simulink library "formationFlyingBlockset"  (R2016b)
settings: Solver=ode45  StartTime=0.0  StopTime=10.0  RelTol=1e-3  EnableMultiTasking=on
undefined symbols (not defined in the file or in its folder): adaptive, aircraftmask_ID, aircraftmask_navigationLaw, aircraftmask_originNED_ECEF_rrm, aircraftmask_p0_NED_m, aircraftmask_phithetapsi_trim, aircraftmask_wakevortexenabled, airkraftmask_displayLeader, DiscIntNeverNeededParam, Earth, fflib_degdegm2rrm, fflib_Hz2radps, fflib_rrm2degdegm, flat2lla, hinf, Klqr, lquadr, mask_ac, mask_ID, mpc, poleplacement, uavsim, washout, WGS84
undefined symbols (not defined in the file): aircraftmask_phithetapsi0, aircraftmask_pqr0, aircraftmask_uvw0, innerloop, outerloop, tatestos
libraries: formationFlyingBlockset x59, aerolibtransform2 x42, simulink_extras x27, dspsrcs4 x11, aerolibutil x5, uavsimBlockset_UAV3DInterface x4, uavsimBlockset_ServoHS55 x4, uavsimBlockset_VectorNorm x3, uavsimBlockset_UAV3DVisualization x3, uavsimBlockset_AugmentWind x3, stringquartett x2, Parrot_DCAS_lib x2
(part 2 of 5)

== system formationFlyingBlockset/Parrot drone ==
  Environment : Inport  OutDataTypeStr=Bus: Environment
  Bus Creator : BusCreator  Inputs=2  OutDataTypeStr=Bus: iUAScom
  Bus Creator1 : BusCreator  Inputs=1  OutDataTypeStr=Bus: FlightGearData  NonVirtualBus=on
  Bus Selector1 : BusSelector  OutputSignals=Kinematics.Position.P_NED_m,Kinematics.Velocity.Vground_NED_mps
  Constant : Constant  Value=zeros(6,1)
  Gain : Gain
  Gain1 : Gain
  ID : Constant  Value=aircraftmask_ID
  MATLAB Function : MATLAB Function  TreatAsAtomicUnit=on
  No Elevation model : Constant  Value=0
  Parrot drone open loop dynamics : formationFlyingBlockset/Parrot drone open loop dynamics  mask_phithetapsi0=aircraftmask_phithetapsi0  mask_p0_ECEF_lla=fflib_degdegm2rrm(flat2lla(aircraftmask_p0_NED_m, rad2deg(aircraftmask_originNED_ECEF_rrm(1:2)), 0, aircraftmask_originNED_ECEF_rrm(3)))  mask_originNED_ECEF_rrm=aircraftmask_originNED_ECEF_rrm  mask_pqr0=aircraftmask_pqr0  mask_uvw0=aircraftmask_uvw0  uavsim=uavsim
  Simulation Time : formationFlyingBlockset/Signal to workspace  mask_id=['log_machinetime_UAS' num2str(aircraftmask_ID) ]  mask_dt=1  mask_debug=log_machinetime_UAS1
  Terminator5 : Terminator
  UAV3D Visualization : uavsimBlockset_UAV3DVisualization/UAV3D Visualization  mask_visual=3
  control surface deflections : formationFlyingBlockset/Signal to workspace  mask_id=['log_csdeflct_UAS' num2str(aircraftmask_ID) ]  mask_dt=-1  mask_debug=log_csdeflct_UAS1
  AirframeBus : Outport
  Grounddata : Outport  Port=2  OutDataTypeStr=Bus: FlightGearData
  iUASCom out : Outport  Port=3
  wires:
  MATLAB Function/1(t) -> Simulation Time/1
  Bus Creator/1 -> iUASCom out/1
  Bus Selector1/2 -> Gain/1  "<Vground_NED_mps>"
  Bus Selector1/1 -> Gain1/1  "<P_NED_m>"
  Gain1/1 -> Bus Creator/1  "P_NED_m"
  Gain/1 -> Bus Creator/2  "Vground_NED_mps"
  Constant/1 -> Parrot drone open loop dynamics/3
  Parrot drone open loop dynamics/3 -> control surface deflections/1, UAV3D Visualization/3
  Parrot drone open loop dynamics/1 -> Bus Selector1/1, AirframeBus/1, UAV3D Visualization/1
  Environment/1 -> Parrot drone open loop dynamics/2
  ID/1 -> UAV3D Visualization/2
  Bus Creator1/1 -> Grounddata/1
  No Elevation model/1 -> Bus Creator1/1  "groundlevel_NED_m"
  UAV3D Visualization/1 -> Terminator5/1

== system formationFlyingBlockset/Parrot drone open loop dynamics ==
  u - system inputs : Inport  OutDataTypeStr=Bus: CMD_quadrotor
  Environment : Inport  Port=2  OutDataTypeStr=Bus: Environment
  External forces and moments : Inport  Port=3
  Vehicle model : Subsystem
  Airframe : Outport  OutDataTypeStr=Bus: Airframe
  C_aero_w : Outport  Port=2
  effective commands : Outport  Port=3  OutDataTypeStr=Bus: CMD_quadrotor
  FMprop : Outport  Port=4
  wires:
  Environment/1 -> Vehicle model/2(EnvData)
  Vehicle model/2(Cwind) -> C_aero_w/1
  External forces and moments/1 -> Vehicle model/3(FM_external)
  u - system inputs/1 -> Vehicle model/1(CMD), effective commands/1
  Vehicle model/1(Airframe) -> Airframe/1
  Vehicle model/3(FMprop) -> FMprop/1

== system formationFlyingBlockset/Quadcopter avionics ==
  inter UAS com : Inport  OutDataTypeStr=Bus: iUAScom
  formation delta_p : Inport  Port=2
  true aircraft state : Inport  Port=3
  Environment : Inport  Port=4  OutDataTypeStr=Bus: Environment
  P propulsion : Inport  Port=5
  fstate_dx_in : Inport  Port=6
  vLeaderState : Inport  Port=7  OutDataTypeStr=Bus: iUAScom
  Add sensor errors : formationFlyingBlockset/Add sensor errors
  Bus Selector : BusSelector  OutputSignals=Kinematics.Position.P_NED_m,Kinematics.Velocity.Vground_NED_mps,Kinematics.Acceleration.VgroundDot_bfrozen_mps2,Kinematics.Attitude.DCM_be
  Command laws - code generation - : Subsystem  TreatAsAtomicUnit=on  SystemSampleTime=0.01
  Display : Display
  Math Function : Math  Operator=transpose  SaturateOnIntegerOverflow=on
  Matrix Multiply : Product  Multiplication=Matrix(*)
  NED acceleration : formationFlyingBlockset/Signal to workspace  mask_id=['log_accNED_UAS' num2str(aircraftmask_ID) ]  mask_dt=0.01  mask_debug=log_accNED_UAS1
  NED position : formationFlyingBlockset/Signal to workspace  mask_id=['log_pNED_UAS' num2str(aircraftmask_ID) ]  mask_dt=0.1  mask_debug=log_pNED_UAS1
  NED velocity : formationFlyingBlockset/Signal to workspace  mask_id=['log_vNED_UAS' num2str(aircraftmask_ID) ]  mask_dt=0.1  mask_debug=log_vNED_UAS1
  PWM+computation delay : Delay  DelayLength=ceil(uavsim.avionics.totaltransportdelay_s/(1/uavsim.simConfig.sampleFrequency))
  Perfect Sensors : formationFlyingBlockset/Perfect Sensors
  Propulsion power : formationFlyingBlockset/Signal to workspace  mask_id=['log_P_propulsion_UAS' num2str(aircraftmask_ID) ]  mask_dt=0.1  mask_debug=log_P_propulsion_UAS1
  Sensor delays1 : Subsystem  Commented=on
  Sensor error models on/off : ManualSwitch
  Sensor log : formationFlyingBlockset/Signal to workspace  mask_id=['log_sensors_UAS' num2str(aircraftmask_ID) ]  mask_dt=0.01  mask_debug=log_sensors_UAS1
  Sensor log - error-free : formationFlyingBlockset/Signal to workspace  mask_id=['log_cleansensors_UAS' num2str(aircraftmask_ID) ]  mask_dt=0.01  mask_debug=log_cleansensors_UAS1
  State estimation department : formationFlyingBlockset/State estimation department
  u : Outport
  fstate_dx : Outport  Port=2
  wires:
  fstate_dx_in/1 -> ?
  ? -> fstate_dx/1
  Perfect Sensors/1 -> Add sensor errors/1, Sensor error models on/off/1, Sensor log - error-free/1
  Bus Selector/2 -> Display/1, NED velocity/1  "<Vground_NED_mps>"
  Bus Selector/1 -> NED position/1  "<P_NED_m>"
  true aircraft state/1 -> Perfect Sensors/1, Bus Selector/1
  P propulsion/1 -> Propulsion power/1
  Environment/1 -> Perfect Sensors/3
  State estimation department/1 -> Command laws - code generation -/1(Aircraft state estimate)
  inter UAS com/1 -> Perfect Sensors/2
  formation delta_p/1 -> ?
  PWM+computation delay/1 -> u/1
  Command laws - code generation -/1(u - system inputs) -> PWM+computation delay/1
  Bus Selector/4 -> Math Function/1  "<DCM_be>"
  Bus Selector/3 -> Matrix Multiply/2  "<VgroundDot_bfrozen_mps2>"
  Math Function/1 -> Matrix Multiply/1
  Matrix Multiply/1 -> NED acceleration/1
  Sensor error models on/off/1 -> State estimation department/1, Sensor log/1
  Add sensor errors/1 -> Sensor error models on/off/2
  vLeaderState/1 -> ?

== system formationFlyingBlockset/Rotation: planar leader speed frame to NED frame ==
  v of planar frame reference velocity in NED [mps] : Inport
  r planar speed frame : Inport  Port=2
  Constant : Constant  Value=zeros(1,1)
  Constant1 : Constant  Value=zeros(1,1)
  Demux : Demux  Outputs=3
  Math Function : Math  Operator=transpose  SaturateOnIntegerOverflow=on
  Mux : Mux  Inputs=3
  Rotate vector : Product  Multiplication=Matrix(*)
  Rotation Angles to Direction Cosine Matrix : aerolibtransform2/Rotation Angles to Direction Cosine Matrix  rotationOrder=ZYX
  Trigonometric Function : Trigonometry  Operator=atan2
  r NED : Outport
  wires:
  Rotation Angles to Direction Cosine Matrix/1 -> Math Function/1
  Demux/1 -> Trigonometric Function/2
  Demux/2 -> Trigonometric Function/1
  r planar speed frame/1 -> Rotate vector/2
  Trigonometric Function/1 -> Mux/1  "psi"
  Mux/1 -> Rotation Angles to Direction Cosine Matrix/1
  Constant/1 -> Mux/3  "phi"
  Rotate vector/1 -> r NED/1
  v of planar frame reference velocity in NED [mps]/1 -> Demux/1
  Constant1/1 -> Mux/2  "theta"
  Math Function/1 -> Rotate vector/1

== system formationFlyingBlockset/Sensor package: error-free ==
  aircraft state : Inport  OutDataTypeStr=Bus: Airframe
  inter UAS com : Inport  Port=2  OutDataTypeStr=Bus: iUAScom
  Environment : Inport  Port=3  OutDataTypeStr=Bus: Environment
  AHRS : Subsystem
  Air Data : Subsystem
  Bus Object Bus Creator : BusCreator  Inputs=8  OutDataTypeStr=Bus: SensorBus  mask(BUS OBJECT Bus Creator){busType=Bus: SensorBus}
      mask prompts: busType "Bus Type"
      mask help:
      | Provides users the cabability to painlessly, instantly customize bus creators of output data type 'Bus:' by selecting the bus object type from a drop down menu dynamically populated by bus objects in the workspace.
      |
      | After pressing the "Apply Selection" button signal lines into the creator are populated and named with the elements in the chosen bus saving the user from having to recall and fill out signal line names.
      |
      | NOTE that when copying a Bus Object Bus Creator from your locked Library the link to the Library is automatically broken. This saves the user from having to Unlock Links To Library (From the Library menu.), Disable Link and finally Break Link (Both from the Model menu.) for every placed instance of the block.
      settings: AttributesFormatString=%<OutDataTypeStr>  CopyFcn=set_param(gcb, 'LinkStatus', 'none')
      mask TypeOptions busType: Bus: AHRS | Bus: Acceleration | Bus: Aero | Bus: Airdata | Bus: Airframe | Bus: Attitude | Bus: CMD | Bus: CMD_quadrotor | Bus: ControlInfoBus | Bus: Enginedata | Bus: Environment | Bus: FlightGearData | Bus: GCSUpstream | Bus: GNSSL1 | Bus: GNSSRTK | Bus: GPS | Bus: IMU | Bus: Kinematics | Bus: LandinggearInput | Bus: MotionTracker | Bus: Position | Bus: Radiodistance | Bus: RotationalAcceleration | Bus: RotationalVelocity | Bus: SensorBus | Bus: StateBus | Bus: Velocity | Bus: WindAngles | Bus: iUAScom
      mask Callback busType:
      | % Using variable names terminated with "_BOBC" to lessen the chances of
      | % collisions with existing workspace variables.
      | 
      | % Get the current block handle and mask handle.
      | handleCreator_BOBC = gcbh;
      | maskObj_BOBC       = Simulink.Mask.get(gcb);
      | 
      | % Get a list of variables in the workspace in order to search for the '1x1
      | % Bus' types.
      | wsVars_BOBC = whos;
      | 
      | % Reset the 'TypeOptions' bus list in case some '1x1 Bus' types have been
      | % deleted from or added to the workspace.
      | maskObj_BOBC.Parameters.TypeOptions = {'<empty>'};
      | 
      | % Reset the bus count.
      | busCount_BOBC = 0;
      | 
      | for index_BOBC = 1:length(wsVars_BOBC)
      | 
      |    % If the variable is a bus object...
      |    if strcmp(wsVars_BOBC(index_BOBC).class, 'Simulink.Bus')
      | 
      |       busCount_BOBC = busCount_BOBC + 1;
      | 
      |       % ... add it to the TypeOptions of the mask.
      |       maskObj_BOBC.Parameters.TypeOptions(busCount_BOBC) = ...
      |                                                            ...
      |                                  {['Bus: ', wsVars_BOBC(index_BOBC).name]};
      |    end
      | end
      | 
      | if busCount_BOBC == 0
      | 
      |    % If there are NO bus objects in the workspace then provide a warning
      |    % popup...
      |    warndlg('There are currently no bus objects in the workspace - you have no use for this block. Use a normal Bus Creator instead.')
      | 
      |    % ... and do nothing.
      | elseif ~strcmp(get_param(handleCreator_BOBC, 'OutDataTypeStr'), 'Inherit: auto')
      | 
      |    % If the currently selected bus data type ('OutDataTypeStr') is not
      |    % 'Inherit: auto' (i.e., if we are reopening the mask.) then get the
      |    % current 'OutDataTypeStr' and 'maskVal.' ('maskVal' is the selected
      |    % 'TypeOptions' list member.)
      |    outDatStr_BOBC = get_param(handleCreator_BOBC, 'OutDataTypeStr');
      |    maskVal_BOBC   = get_param(handleCreator_BOBC, 'MaskValues');
      | 
      |    if ~strcmp(outDatStr_BOBC, maskVal_BOBC{1})
      | 
      |       % Upon re-opening the mask if the default 'TypeOptions' list member
      |       % (The first one.) contained in 'maskVal' does not match the
      |       % currently selected bus data type ('OutDataTypeStr') then set the
      |       % 'TypeOptions' list member to the selected bus data type. (Cuts down
      |       % on confusion to have the displayed list member match the selected
      |       % bus data type rather than the first entry.)
      |       set_param(handleCreator_BOBC, 'MaskValues', {outDatStr_BOBC});
      |    end
      | end
      | 
      | % Clean up the workspace.
      | clear  handleCreator_BOBC  maskObj_BOBC     wsVars_BOBC ...
      |             busCount_BOBC    index_BOBC  outDatStr_BOBC ...
      |              maskVal_BOBC
      mask DialogControl applyMOCBSelection Prompt: Apply Selection
      mask DialogControl applyMOCBSelection Callback:
      | % Using variable names terminated with "_BOBC" to lessen the chances of
      | % collisions with existing workspace variables.
      | 
      | % Get the current block, current block handle and mask handle.
      | currentBlock_BOBC  = gcb;
      | handleCreator_BOBC = gcbh;
      | 
      | % Get the desired bus type...
      | desiredBusType_BOBC = get_param(handleCreator_BOBC, 'busType');
      | 
      | % ... and set the 'OutDataTypeStr' to it.
      | set_param(handleCreator_BOBC, 'OutDataTypeStr', desiredBusType_BOBC);
      | 
      | %% First delete any existing lines on the port.
      | % Get the line handles.
      | lh_BOBC = get_param(handleCreator_BOBC, 'LineHandles');
      | 
      | % If any lines exist (Non- -1 line handles.), delete them and start over.
      | if max(lh_BOBC.Inport > 0)
      | 
      |    for index_BOBC = 1:length(lh_BOBC.Inport)
      | 
      |       if lh_BOBC.Inport(index_BOBC) > 0
      | 
      |          delete_line(lh_BOBC.Inport(index_BOBC))
      |       end
      |    end
      | end
      | 
      | %% Then work on adding new lines.
      | 
      | % Get the block path for 'add_line' function.
      | blockPath_BOBC = get_param(handleCreator_BOBC, 'Parent');
      | 
      | % Get the newly selected bus type ('OutDataTypeStr')...
      | mocbBusType_BOBC = get_param(currentBlock_BOBC, 'OutDataTypeStr');
      | 
      | % ... and parse off "Bus: " so the string of the desired bus contained in
      | % 'OutDataTypeStr' matches the raw workspace bus names.
      | mocbBusType_BOBC = mocbBusType_BOBC(6:end);
      | 
      | % Then evaluate the string containing the workspace bus name which will
      | % load the desired bus parameters.
      | busParams_BOBC = eval(mocbBusType_BOBC);
      | 
      | % From the parameters grab the number of lines to add.
      | numLines_BOBC = length(busParams_BOBC.Elements);
      | 
      | % Set the number of inputs of the masked bus creator to the number of lines
      | % to add.
      | set_param(handleCreator_BOBC, 'Inputs', num2str(numLines_BOBC));
      | 
      | % Get (Inputs.) port handles so we can grab the positions of them.
      | ph_BOBC = get_param(handleCreator_BOBC, 'PortHandles');
      | 
      | for index_BOBC = 1:numLines_BOBC
      | 
      |    % Get the position of input port number 'index_BOBC'.
      |    portPos_BOBC = get_param(ph_BOBC.Inport(index_BOBC), 'Position');
      | 
      |    % Add a line from 50 pixels left of the port position to the port
      |    % position. (This must be done because it's the lines that get named,
      |    % not the port positions.)
      |    portLine_BOBC = add_line(blockPath_BOBC, [portPos_BOBC - [50 0]; portPos_BOBC]);
      | 
      |    % Rename the new line to the bus 'index_BOBC-st/nd/rd/th' element name.
      |    set_param(portLine_BOBC, 'Name', busParams_BOBC.Elements(index_BOBC).Name)
      | end
      | 
      | %% Cleanup the workspace.
      | clear    currentBlock_BOBC  handleCreator_BOBC      index_BOBC ...
      |        desiredBusType_BOBC             lh_BOBC  blockPath_BOBC ...
      |           mocbBusType_BOBC      busParams_BOBC   numLines_BOBC ...
      |                    ph_BOBC        portPos_BOBC   portLine_BOBC
  L1 GPS : Subsystem
  Optitrack : Subsystem
  Propulsion sensors : Subsystem
  RTK DGPS : Subsystem
  Radio distance sensor : Subsystem
  Wind angle sensors : Subsystem
  sensor readings : Outport
  wires:
  Environment/1 -> AHRS/2(Environment)
  aircraft state/1 -> Air Data/1(aircraft state), Wind angle sensors/1(aircraft state), Optitrack/1(aircraft state), Propulsion sensors/1(aircraft state), Radio distance sensor/1(aircraft state), RTK DGPS/1(aircraft state), L1 GPS/1(aircraft state), AHRS/1(aircraft state)
  inter UAS com/1 -> RTK DGPS/2(inter UAS com), Radio distance sensor/2(inter UAS com)
  Bus Object Bus Creator/1 -> sensor readings/1
  AHRS/1(output) -> Bus Object Bus Creator/1  "ahrs"
  Air Data/1(output) -> Bus Object Bus Creator/2  "airdata"
  L1 GPS/1(output) -> Bus Object Bus Creator/3  "gnss_l1"
  RTK DGPS/1(output) -> Bus Object Bus Creator/4  "gnss_rtk"
  Propulsion sensors/1(output) -> Bus Object Bus Creator/5  "propulsion"
  Radio distance sensor/1(output) -> Bus Object Bus Creator/6  "radiodistance"
  Wind angle sensors/1(output) -> Bus Object Bus Creator/7  "windangles"
  Optitrack/1(output) -> Bus Object Bus Creator/8  "motiontracker"

== system formationFlyingBlockset/Signal to workspace ==
  In : Inport
  log_ucontroller_UAS1 : ToWorkspace  VariableName=log_ucontroller_UAS1  SaveFormat=Timeseries  SampleTime=mask_dt
  wires:
  In/1 -> log_ucontroller_UAS1/1

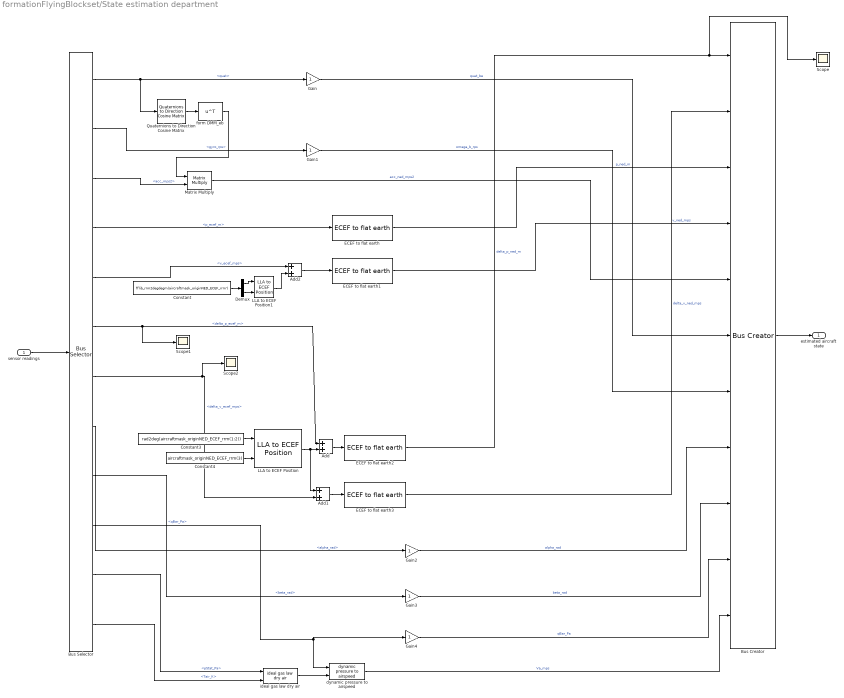
== system formationFlyingBlockset/State estimation department ==
  sensor readings : Inport  OutDataTypeStr=Bus: SensorBus
  Add : Sum
  Add1 : Sum
  Add2 : Sum
  Bus Creator : BusCreator  Inputs=11  OutDataTypeStr=Bus: StateBus
  Bus Selector : BusSelector  OutputSignals=ahrs.quat,ahrs.gyro_rps,ahrs.acc_mps2,gnss_l1.p_ecef_m,gnss_l1.v_ecef_mps,gnss_rtk.delta_p_ecef_m,gnss_rtk.delta_v_ecef_mps,windangles.alpha_rad,windangles.beta_rad,airdata.qBar_Pa,airdata.pStat_Pa,airdata.Tair_K
  Constant : Constant  Value=fflib_rrm2degdegm(aircraftmask_originNED_ECEF_rrm')
  Constant3 : Constant  Value=rad2deg(aircraftmask_originNED_ECEF_rrm(1:2))
  Constant4 : Constant  Value=aircraftmask_originNED_ECEF_rrm(3)
  Demux : Demux  Outputs=[2 1]
  ECEF to flat earth{,1..3} (4 alike) : formationFlyingBlockset/ECEF to flat earth  mask_originNED_ECEF_rrm=aircraftmask_originNED_ECEF_rrm
  Gain{,1..4} (5 alike) : Gain
  LLA to ECEF Position : aerolibtransform2/LLA to ECEF Position  units=Metric (MKS)  ptype=Earth (WGS84)  F=1/298.257223563  R=6378137
  LLA to ECEF Position1 : aerolibtransform2/LLA to ECEF Position  units=Metric (MKS)  ptype=Earth (WGS84)  F=1/298.257223563  R=6378137
  Matrix Multiply : Product  Multiplication=Matrix(*)
  Quaternions to Direction Cosine Matrix : aerolibtransform2/Quaternions to  Direction Cosine Matrix
  Scope : Scope
  Scope1 : Scope
  Scope2 : Scope
  dynamic pressure to airspeed : formationFlyingBlockset/dynamic pressure to airspeed
  form DMM_eb : Math  Operator=transpose  SaturateOnIntegerOverflow=on
  ideal gas law dry air : formationFlyingBlockset/ideal gas law dry air
  estimated aircraft state : Outport  OutDataTypeStr=Bus: StateBus
  wires:
  sensor readings/1 -> Bus Selector/1
  Bus Creator/1 -> estimated aircraft state/1
  Bus Selector/1 -> Quaternions to Direction Cosine Matrix/1, Gain/1  "<quat>"
  Bus Selector/2 -> Gain1/1  "<gyro_rps>"
  Bus Selector/3 -> Matrix Multiply/2  "<acc_mps2>"
  Bus Selector/4 -> ECEF to flat earth/1  "<p_ecef_m>"
  Bus Selector/6 -> Add/1, Scope1/1  "<delta_p_ecef_m>"
  Bus Selector/7 -> Add1/2, Scope2/1  "<delta_v_ecef_mps>"
  Bus Selector/8 -> Gain2/1  "<alpha_rad>"
  Bus Selector/9 -> Gain3/1  "<beta_rad>"
  ECEF to flat earth2/1 -> Bus Creator/1, Scope/1  "delta_p_ned_m"
  ECEF to flat earth3/1 -> Bus Creator/2  "delta_v_ned_mps"
  ECEF to flat earth/1 -> Bus Creator/3  "p_ned_m"
  ECEF to flat earth1/1 -> Bus Creator/4  "v_ned_mps"
  Matrix Multiply/1 -> Bus Creator/5  "acc_ned_mps2"
  form DMM_eb/1 -> Matrix Multiply/1
  Quaternions to Direction Cosine Matrix/1 -> form DMM_eb/1
  Constant3/1 -> LLA to ECEF Position/1
  Constant4/1 -> LLA to ECEF Position/2
  LLA to ECEF Position/1 -> Add1/1, Add/2
  Gain/1 -> Bus Creator/6  "quat_be"
  Gain1/1 -> Bus Creator/7  "omega_b_rps"
  Gain2/1 -> Bus Creator/8  "alpha_rad"
  Gain3/1 -> Bus Creator/9  "beta_rad"
  Bus Selector/10 -> dynamic pressure to airspeed/1, Gain4/1  "<qBar_Pa>"
  Gain4/1 -> Bus Creator/10  "qBar_Pa"
  Bus Selector/11 -> ideal gas law dry air/1  "<pStat_Pa>"
  Bus Selector/12 -> ideal gas law dry air/2  "<Tair_K>"
  ideal gas law dry air/1 -> dynamic pressure to airspeed/2
  dynamic pressure to airspeed/1 -> Bus Creator/11  "Va_mps"
  Bus Selector/5 -> Add2/1  "<v_ecef_mps>"
  Constant/1 -> Demux/1
  Demux/1 -> LLA to ECEF Position1/1
  Demux/2 -> LLA to ECEF Position1/2
  LLA to ECEF Position1/1 -> Add2/2
  Add2/1 -> ECEF to flat earth1/1
  Add1/1 -> ECEF to flat earth3/1
  Add/1 -> ECEF to flat earth2/1

== system formationFlyingBlockset/UAV3D Visualization ==
  ID : Inport
  CMD : Inport  Port=2  OutDataTypeStr=Bus: CMD
  p_NED_m : Inport  Port=3
  DCM_be : Inport  Port=4
  Bus Selector2 : BusSelector  OutputSignals=da_rad,de_rad,dr_rad,den_0to1,df_rad
  Demux : Demux  Outputs=3
  Demux1 : Demux
  Direction Cosine Matrix to Quaternions : aerolibtransform2/Direction Cosine Matrix  to Quaternions
  ID1 : Constant  Value=mask_visual-1
  UAV3D interface : uavsimBlockset_UAV3DInterface/UAV3D interface  ip='localhost'  udpport=4445
  wires:
  ID1/1 -> UAV3D interface/14
  ID/1 -> UAV3D interface/1
  Direction Cosine Matrix to Quaternions/1 -> Demux1/1
  Demux1/4 -> UAV3D interface/8
  Demux1/3 -> UAV3D interface/7
  Demux1/2 -> UAV3D interface/6
  Demux1/1 -> UAV3D interface/5
  DCM_be/1 -> Direction Cosine Matrix to Quaternions/1
  Demux/1 -> UAV3D interface/2
  Demux/2 -> UAV3D interface/3
  Demux/3 -> UAV3D interface/4
  p_NED_m/1 -> Demux/1
  CMD/1 -> Bus Selector2/1
  Bus Selector2/1 -> UAV3D interface/9  "<da_rad>"
  Bus Selector2/2 -> UAV3D interface/10  "<de_rad>"
  Bus Selector2/3 -> UAV3D interface/11  "<dr_rad>"
  Bus Selector2/4 -> UAV3D interface/12  "<den_0to1>"
  Bus Selector2/5 -> UAV3D interface/13  "<df_rad>"

== system formationFlyingBlockset/UAV3D Visualization1 ==
  ID : Inport
  pNED : Inport  Port=2
  q_be : Inport  Port=3
  Constant : Constant
  Demux : Demux  Outputs=3
  Demux1 : Demux
  ID1 : Constant  Value=mask_visual-1
  UAV3D interface : uavsimBlockset_UAV3DInterface/UAV3D interface  ip='localhost'  udpport=4445
  wires:
  pNED/1 -> Demux/1
  Demux/3 -> UAV3D interface/4
  Demux/2 -> UAV3D interface/3
  Demux/1 -> UAV3D interface/2
  Demux1/1 -> UAV3D interface/5
  Demux1/2 -> UAV3D interface/6
  Demux1/3 -> UAV3D interface/7
  Demux1/4 -> UAV3D interface/8
  q_be/1 -> Demux1/1
  ID/1 -> UAV3D interface/1
  ID1/1 -> UAV3D interface/14
  Constant/1 -> UAV3D interface/Enable

== system formationFlyingBlockset/Virtual leader ==
  Bus Creator : BusCreator  Inputs=2  OutDataTypeStr=Bus: iUAScom
  Clock : Clock
  Gain : Gain
  Gain1 : Gain
  MATLAB Function : MATLAB Function  TreatAsAtomicUnit=on
  Scope : Scope
  Virtual leader ID : Constant  Value=300  VectorParams1D=off
  Visualize NED position : formationFlyingBlockset/Visualize leader  mask_3dmodel=3
  iUASCom out : Outport
  FormationLeaderState : Outport  Port=2
  wires:
  Virtual leader ID/1 -> Visualize NED position/3
  Clock/1 -> MATLAB Function/1(t_UTC_s)
  Bus Creator/1 -> iUASCom out/1, FormationLeaderState/1
  MATLAB Function/2(vLeader_NED_mps) -> Gain/1, Visualize NED position/2
  MATLAB Function/1(pLeader_NED_m) -> Gain1/1, Visualize NED position/1, Scope/1
  Gain1/1 -> Bus Creator/1  "P_NED_m"
  Gain/1 -> Bus Creator/2  "Vground_NED_mps"

== system formationFlyingBlockset/Visualize leader ==
  p_NED_m : Inport
  v_NED_mps : Inport  Port=2
  ID : Inport  Port=3
  3D model : Constant  Value=mask_3dmodel
  Always enabled : Constant
  Compute chi : Trigonometry  Operator=atan2
  Constant : Constant  Value=0
  Constant2 : Constant  Value=zeros(2,1)
  Demux : Demux  Outputs=3
  Demux1 : Demux
  Mux : Mux  Inputs=2
  Rotation Angles to Quaternions : aerolibtransform2/Rotation Angles to Quaternions  rotationOrder=ZYX
  UAV3D interface : uavsimBlockset_UAV3DInterface/UAV3D interface  ip='localhost'  udpport=4445
  get vx : Selector  InputPortWidth=3  IndexOptions=Index vector (dialog)  Indices=1  OutputSizes=1
  get vy : Selector  InputPortWidth=3  IndexOptions=Index vector (dialog)  Indices=2  OutputSizes=1
  wires:
  Always enabled/1 -> UAV3D interface/Enable
  3D model/1 -> UAV3D interface/14
  ID/1 -> UAV3D interface/1
  Constant/1 -> UAV3D interface/9, UAV3D interface/10, UAV3D interface/11, UAV3D interface/12, UAV3D interface/13
  Demux1/3 -> UAV3D interface/7
  Compute chi/1 -> Mux/1
  Rotation Angles to Quaternions/1 -> Demux1/1
  Mux/1 -> Rotation Angles to Quaternions/1
  Constant2/1 -> Mux/2
  v_NED_mps/1 -> get vx/1, get vy/1
  get vx/1 -> Compute chi/2
  get vy/1 -> Compute chi/1
  p_NED_m/1 -> Demux/1
  Demux1/4 -> UAV3D interface/8
  Demux1/2 -> UAV3D interface/6
  Demux1/1 -> UAV3D interface/5
  Demux/3 -> UAV3D interface/4
  Demux/2 -> UAV3D interface/3
  Demux/1 -> UAV3D interface/2

== system formationFlyingBlockset/Visualize vortex tunnel in UAV3D ==
  ID : Inport
  p_NED_m : Inport  Port=2
  transparency [0,1] : Inport  Port=3
  length_m : Inport  Port=4
  radius_m : Inport  Port=5
  dcm_ew : Inport  Port=6
  enable UDP : Inport  Port=7
  Demux : Demux  Outputs=3
  Demux1 : Demux
  Direction Cosine Matrix to Quaternions : aerolibtransform2/Direction Cosine Matrix  to Quaternions
  ID1 : Constant  Value=7
  ID2 : Constant  Value=0
  Math Function : Math  Operator=transpose  SaturateOnIntegerOverflow=on
  UAV3D interface : uavsimBlockset_UAV3DInterface/UAV3D interface  ip='localhost'  udpport=4445
  wires:
  enable UDP/1 -> UAV3D interface/Enable
  Math Function/1 -> Direction Cosine Matrix to Quaternions/1
  Direction Cosine Matrix to Quaternions/1 -> Demux1/1
  ID2/1 -> UAV3D interface/11, UAV3D interface/13
  radius_m/1 -> UAV3D interface/10
  length_m/1 -> UAV3D interface/9
  p_NED_m/1 -> Demux/1
  dcm_ew/1 -> Math Function/1
  ID/1 -> UAV3D interface/1
  ID1/1 -> UAV3D interface/14
  Demux1/4 -> UAV3D interface/8
  Demux1/3 -> UAV3D interface/7
  Demux1/2 -> UAV3D interface/6
  Demux/3 -> UAV3D interface/4
  Demux/1 -> UAV3D interface/2
  Demux/2 -> UAV3D interface/3
  Demux1/1 -> UAV3D interface/5
  transparency [0,1]/1 -> UAV3D interface/12

== system formationFlyingBlockset/Wake vortex effects ==
  AirframeBus : Inport  OutDataTypeStr=Bus: Airframe
  Environment : Inport  Port=2  OutDataTypeStr=Bus: Environment
  Ci_w : Inport  Port=3
  enable UAV3D : Inport  Port=4
  Augment atmospheric wind and wind gradients by induced wind and effects of induced wind gradients : uavsimBlockset_AugmentWind/Augment atmospheric wind and wind gradients by induced wind and induced wind gradients
  Constant : Constant  Value=aircraftmask_wakevortexenabled
  Constant1 : Constant  Value=zeros(3,1)
  Constant2 : Constant  Value=zeros(3,1)
  If : If  IfExpression=u1 ~= 0
  Subsystem : Subsystem
  Switch : Switch  Criteria=u2 ~= 0
  Switch1 : Switch  Criteria=u2 ~= 0
  Terminator : Terminator
  Visualize vortices in UAV3D : Subsystem
  EnvData_augmented : Outport  OutDataTypeStr=Bus: Environment
  wires:
  AirframeBus/1 -> Subsystem/1(AirframeBus)
  Constant/1 -> Switch/2, Switch1/2, If/1
  Ci_w/1 -> Subsystem/2(Ci_w)
  Environment/1 -> Augment atmospheric wind and wind gradients by induced wind and effects of induced wind gradients/1
  Subsystem/1(Vi_bfrozen) -> Switch/1
  Subsystem/2(omegai_bfrozen) -> Switch1/1
  Constant1/1 -> Switch/3
  Switch/1 -> Augment atmospheric wind and wind gradients by induced wind and effects of induced wind gradients/2
  Switch1/1 -> Augment atmospheric wind and wind gradients by induced wind and effects of induced wind gradients/3
  Constant2/1 -> Switch1/3
  Augment atmospheric wind and wind gradients by induced wind and effects of induced wind gradients/1 -> EnvData_augmented/1
  If/1 -> Subsystem/Action
  If/2 -> Terminator/1
  Subsystem/3(vortex parameters) -> Visualize vortices in UAV3D/1(vortex parameters)
  enable UAV3D/1 -> Visualize vortices in UAV3D/2(enable UAV3D)

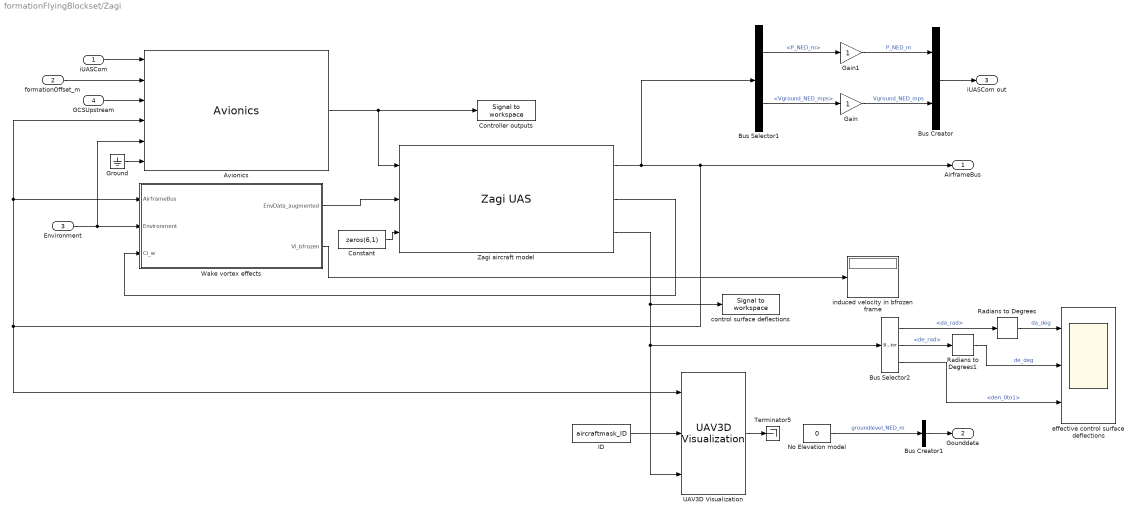
== system formationFlyingBlockset/Zagi ==
  iUASCom : Inport  OutDataTypeStr=Bus: iUAScom
  formationOffset_m : Inport  Port=2
  Environment : Inport  Port=3  OutDataTypeStr=Bus: Environment
  GCSUpstream : Inport  Port=4  OutDataTypeStr=Bus: GCSUpstream
  Avionics : formationFlyingBlockset/Avionics  mask_ac=uavsim.zagi
  Bus Creator : BusCreator  Inputs=2  OutDataTypeStr=Bus: iUAScom
  Bus Creator1 : BusCreator  Inputs=1  OutDataTypeStr=Bus: FlightGearData  NonVirtualBus=on
  Bus Selector1 : BusSelector  OutputSignals=Kinematics.Position.P_NED_m,Kinematics.Velocity.Vground_NED_mps
  Bus Selector2 : BusSelector  OutputSignals=da_rad,de_rad,den_0to1
  Constant : Constant  Value=zeros(6,1)
  Controller outputs : formationFlyingBlockset/Signal to workspace  mask_id=['log_ucontroller_UAS' num2str(aircraftmask_ID) ]  mask_dt=-1  mask_debug=log_ucontroller_UAS1
  Gain : Gain
  Gain1 : Gain
  Ground : Ground
  ID : Constant  Value=aircraftmask_ID
  No Elevation model : Constant  Value=0
  Radians to Degrees : simulink_extras/Transformations/Radians to Degrees
  Radians to Degrees1 : simulink_extras/Transformations/Radians to Degrees
  Terminator5 : Terminator
  UAV3D Visualization : uavsimBlockset_UAV3DVisualization/UAV3D Visualization  mask_visual=0
  Wake vortex effects : Subsystem  TreatAsAtomicUnit=on
  Zagi aircraft model : uavsimBlockset_ZagiUAS/Zagi UAS  mask_zagi_phithetapsi0=aircraftmask_phithetapsi0  mask_zagi_p0_ECEF_lla=fflib_degdegm2rrm(flat2lla(aircraftmask_p0_NED_m, rad2deg(aircraftmask_originNED_ECEF_rrm(1:2)), 0, aircraftmask_originNED_ECEF_rrm(3)))  mask_zagi_originNED_ECEF_rrm=aircraftmask_originNED_ECEF_rrm  mask_zagi_pqr0=aircraftmask_pqr0  mask_zagi_uvw0=aircraftmask_uvw0  uavsim=uavsim
  control surface deflections : formationFlyingBlockset/Signal to workspace  mask_id=['log_csdeflct_UAS' num2str(aircraftmask_ID) ]  mask_dt=-1  mask_debug=log_csdeflct_UAS1
  effective control surface deflections : Scope  NumInputPorts=3
  induced velocity in bfrozen frame : Display
  AirframeBus : Outport
  Gounddata : Outport  Port=2  OutDataTypeStr=Bus: FlightGearData
  iUASCom out : Outport  Port=3
  wires:
  Ground/1 -> Avionics/6
  Bus Selector2/3 -> effective control surface deflections/3  "<den_0to1>"
  Radians to Degrees1/1 -> effective control surface deflections/2  "de_deg"
  Radians to Degrees/1 -> effective control surface deflections/1  "da_deg"
  Avionics/1 -> Controller outputs/1, Zagi aircraft model/1
  GCSUpstream/1 -> Avionics/3
  formationOffset_m/1 -> Avionics/2
  iUASCom/1 -> Avionics/1
  UAV3D Visualization/1 -> Terminator5/1
  No Elevation model/1 -> Bus Creator1/1  "groundlevel_NED_m"
  Bus Creator1/1 -> Gounddata/1
  Bus Selector2/2 -> Radians to Degrees1/1  "<de_rad>"
  Bus Selector2/1 -> Radians to Degrees/1  "<da_rad>"
  ID/1 -> UAV3D Visualization/2
  Wake vortex effects/1(EnvData_augmented) -> Zagi aircraft model/2
  Wake vortex effects/2(Vi_bfrozen) -> induced velocity in bfrozen frame/1
  Zagi aircraft model/2 -> Wake vortex effects/3(Ci_w)
  Environment/1 -> Wake vortex effects/2(Environment), Avionics/5
  Zagi aircraft model/1 -> Wake vortex effects/1(AirframeBus), Avionics/4, UAV3D Visualization/1, AirframeBus/1, Bus Selector1/1
  Zagi aircraft model/3 -> Bus Selector2/1, UAV3D Visualization/3, control surface deflections/1
  Constant/1 -> Zagi aircraft model/3
  Gain/1 -> Bus Creator/2  "Vground_NED_mps"
  Gain1/1 -> Bus Creator/1  "P_NED_m"
  Bus Selector1/1 -> Gain1/1  "<P_NED_m>"
  Bus Selector1/2 -> Gain/1  "<Vground_NED_mps>"
  Bus Creator/1 -> iUASCom out/1

== system formationFlyingBlockset/Zagi actuators - time behaviour ==
  Law output : Inport  OutDataTypeStr=Bus: CMD
  Bus Creator1 : BusCreator  Inputs=5  OutDataTypeStr=Bus: CMD  NonVirtualBus=on
  Bus Selector : BusSelector  OutputSignals=da_rad,de_rad,dr_rad,den_0to1,df_rad
  First order behaviour : TransferFcn  Denominator=[uavsim.zagi.Tengine 1]
  Mux : Mux  Inputs=2
  Radians to Degrees2 : simulink_extras/Transformations/Radians to Degrees
  Rate Transition : RateTransition  Integrity=off
  Servo HS1 : uavsimBlockset_ServoHS55/Servo HS55  deflectionLimits_rad=[deg2rad(-45) deg2rad(45)]  rateLimit_enabled=on  outputLimit_enabled=on  mask_initialPosition=uavsim.zagi.u0.de
  Servo HS2 : uavsimBlockset_ServoHS55/Servo HS55  deflectionLimits_rad=[deg2rad(-45) deg2rad(45)]  rateLimit_enabled=on  outputLimit_enabled=on  mask_initialPosition=uavsim.zagi.u0.dr
  Servo HS3 : uavsimBlockset_ServoHS55/Servo HS55  deflectionLimits_rad=[deg2rad(-10) deg2rad(90)]  rateLimit_enabled=on  outputLimit_enabled=on  mask_initialPosition=uavsim.zagi.u0.df
  Servo HS55 : uavsimBlockset_ServoHS55/Servo HS55  deflectionLimits_rad=[deg2rad(-45) deg2rad(45)]  rateLimit_enabled=on  outputLimit_enabled=on  mask_initialPosition=uavsim.zagi.u0.da
  Terminator2 : Terminator
  Terminator4 : Terminator
  engine input signal saturation : Saturate  UpperLimit=1  LowerLimit=0
  scaling factor2 : Scope
  Effective plant inputs : Outport  OutDataTypeStr=Bus: CMD
  wires:
  First order behaviour/1 -> Bus Creator1/4  "den_0to1"
  Radians to Degrees2/1 -> scaling factor2/1
  Mux/1 -> Radians to Degrees2/1
  Servo HS3/2 -> Terminator4/1
  Servo HS2/2 -> Terminator2/1
  engine input signal saturation/1 -> Rate Transition/1
  Rate Transition/1 -> First order behaviour/1
  Bus Selector/1 -> Servo HS55/1, Mux/1  "<da_rad>"
  Servo HS55/1 -> Bus Creator1/1, Mux/2  "da_rad"
  Servo HS1/1 -> Bus Creator1/2  "de_rad"
  Servo HS2/1 -> Bus Creator1/3  "dr_rad"
  Bus Selector/2 -> Servo HS1/1  "<de_rad>"
  Bus Selector/3 -> Servo HS2/1  "<dr_rad>"
  Bus Selector/4 -> engine input signal saturation/1  "<den_0to1>"
  Law output/1 -> Bus Selector/1
  Bus Creator1/1 -> Effective plant inputs/1  "CMD"
  Bus Selector/5 -> Servo HS3/1  "<df_rad>"
  Servo HS3/1 -> Bus Creator1/5  "df_rad"

== system formationFlyingBlockset/airspeed to dynamic pressure ==
  Va : Inport
  rho : Inport  Port=2
  Divide : Product  Inputs=**
  Gain : Gain  Gain=0.5
  Math Function : Math  Operator=square  SaturateOnIntegerOverflow=on
  qBar : Outport
  wires:
  Divide/1 -> qBar/1
  rho/1 -> Gain/1
  Va/1 -> Math Function/1
  Math Function/1 -> Divide/1
  Gain/1 -> Divide/2

== system formationFlyingBlockset/decomposed state space system ==
  u : Inport
  Demux : Demux  Outputs=2
  Demux1 : Demux  Outputs=2
  Mux1 : Mux  Inputs=2
  Mux2 : Mux  Inputs=2
  inner loop : StateSpace  A=ss_innerloop.a  B=ss_innerloop.b  C=ss_innerloop.c  D=ss_innerloop.d  X0=0
  outer loop : StateSpace  A=ss_outerloop.a  B=ss_outerloop.b  C=ss_outerloop.c  D=ss_outerloop.d  X0=0
  y : Outport
  wires:
  Demux/2 -> Mux1/2
  Mux2/1 -> inner loop/1
  Mux1/1 -> outer loop/1
  u/1 -> Mux1/1, Mux2/1
  Demux1/1 -> y/1
  inner loop/1 -> Demux/1
  outer loop/1 -> Demux1/1
  Demux1/2 -> Mux2/2

== system formationFlyingBlockset/dynamic pressure to airspeed ==
  qBar : Inport
  rho : Inport  Port=2
  Divide : Product  Inputs=*/
  Gain : Gain  Gain=2
  Sqrt : Sqrt  SaturateOnIntegerOverflow=on
  Va : Outport
  wires:
  Divide/1 -> Sqrt/1
  qBar/1 -> Gain/1
  Gain/1 -> Divide/1
  rho/1 -> Divide/2
  Sqrt/1 -> Va/1

== system formationFlyingBlockset/ideal gas law dry air ==
  p : Inport
  T : Inport  Port=2
  Divide : Product  Inputs=*/
  Product : Product
  R_dryair : Constant  Value=287.058
  rho : Outport
  wires:
  R_dryair/1 -> Product/1
  T/1 -> Product/2
  Product/1 -> Divide/2
  p/1 -> Divide/1
  Divide/1 -> rho/1  "rho"

== system formationFlyingBlockset/quaternion to euler angles (zyx rotation) ==
  q : Inport
  Quaternions to Rotation Angles1 : aerolibtransform2/Quaternions to Rotation Angles  rotationOrder=ZYX
  psithetaphi : Outport
  wires:
  Quaternions to Rotation Angles1/1 -> psithetaphi/1
  q/1 -> Quaternions to Rotation Angles1/1

== system formationFlyingBlockset/rotate NED vector to another frame defined by its NED speed vector and an z axis that is aligned with the NED z axis ==
  v of planar frame reference velocity in NED [mps] : Inport
  r planar speed frame : Inport  Port=2
  Constant : Constant  Value=zeros(1,1)
  Constant1 : Constant  Value=zeros(1,1)
  Demux : Demux  Outputs=3
  Mux : Mux  Inputs=3
  Rotate vector : Product  Multiplication=Matrix(*)
  Rotation Angles to Direction Cosine Matrix : aerolibtransform2/Rotation Angles to Direction Cosine Matrix  rotationOrder=ZYX
  Trigonometric Function : Trigonometry  Operator=atan2
  r NED : Outport
  wires:
  Rotation Angles to Direction Cosine Matrix/1 -> Rotate vector/1
  Demux/1 -> Trigonometric Function/2
  Demux/2 -> Trigonometric Function/1
  r planar speed frame/1 -> Rotate vector/2
  Trigonometric Function/1 -> Mux/1  "psi"
  Mux/1 -> Rotation Angles to Direction Cosine Matrix/1
  Constant/1 -> Mux/3  "phi"
  Rotate vector/1 -> r NED/1
  v of planar frame reference velocity in NED [mps]/1 -> Demux/1
  Constant1/1 -> Mux/2  "theta"

== system formationFlyingBlockset/rotate NED vector to another frame defined by its NED speed vector and no bank angle ==
  v of other frame in NED [mps] : Inport
  r NED : Inport  Port=2
  Constant : Constant  Value=zeros(1,1)
  Demux : Demux  Outputs=3
  Divide : Product  Inputs=*/
  Mux : Mux  Inputs=3
  Rotate velocity vector from NED to LS frame : Product  Multiplication=Matrix(*)
  Rotation Angles to Direction Cosine Matrix : aerolibtransform2/Rotation Angles to Direction Cosine Matrix  rotationOrder=ZYX
  Trigonometric Function : Trigonometry  Operator=atan2
  Trigonometric Function1 : Trigonometry  Operator=atan
  r otherframe : Outport
  wires:
  v of other frame in NED [mps]/1 -> Demux/1
  Rotate velocity vector from NED to LS frame/1 -> r otherframe/1
  Constant/1 -> Mux/3  "phi"
  Mux/1 -> Rotation Angles to Direction Cosine Matrix/1
  Trigonometric Function/1 -> Mux/1  "psi"
  r NED/1 -> Rotate velocity vector from NED to LS frame/2
  Demux/2 -> Trigonometric Function/1
  Demux/1 -> Trigonometric Function/2, Divide/2
  Demux/3 -> Divide/1
  Rotation Angles to Direction Cosine Matrix/1 -> Rotate velocity vector from NED to LS frame/1
  Divide/1 -> Trigonometric Function1/1
  Trigonometric Function1/1 -> Mux/2  "theta"

== system formationFlyingBlockset/unit conversion: mps2 to g ==
  "[mps2]" : Inport
  Divide : Product  Inputs=*/
  Standard gravitational acceleration on earth : Constant  Value=9.80665
  "[g]" : Outport
  wires:
  "[mps2]"/1 -> Divide/1
  Divide/1 -> "[g]"/1
  Standard gravitational acceleration on earth/1 -> Divide/2

== system formationFlyingBlockset/v_NED to v_body_frozen ==
  v_NED_mps : Inport
  DCM_be : Inport  Port=2
  Matrix Multiply : Product  Multiplication=Matrix(*)
  v_bfrozen_mps : Outport
  wires:
  Matrix Multiply/1 -> v_bfrozen_mps/1
  v_NED_mps/1 -> Matrix Multiply/2
  DCM_be/1 -> Matrix Multiply/1  "alt_m"

== system formationFlyingBlockset/Add sensor errors/AHRS ==
  perfect sensor reading : Inport  OutDataTypeStr=Bus: SensorBus
  Add noise1 : Sum
  Add noise2 : Sum
  Add noise3 : Sum
  Bus Creator : BusCreator  Inputs=3  OutDataTypeStr=Bus: AHRS
  Bus Selector : BusSelector  OutputSignals=ahrs.quat,ahrs.gyro_rps,ahrs.acc_mps2
  Quaternions to Rotation Angles : aerolibtransform2/Quaternions to Rotation Angles  rotationOrder=ZYX
  Reshape : Reshape
  Reshape1 : Reshape
  Rotation Angles to Quaternions : aerolibtransform2/Rotation Angles to Quaternions  rotationOrder=ZYX
  acceleration noise : dspsrcs4/Random Source  SrcType=Gaussian  NormMethod=Ziggurat  CltLength=12  MinVal=0  MaxVal=1  MeanVal=[0 0 0]'  VarVal=0.01 * [0.0101 0.0116 0.0144]' .^ 2  RepMode=Not repeatable  rawSeed=1  IsInherit=off  SampMode=Discrete  SampTime=1/100  SampFrame=1  DataType=Double  OutComplex=Real  OutputFrames=on
  angular rate noise : dspsrcs4/Random Source  SrcType=Gaussian  NormMethod=Ziggurat  CltLength=12  MinVal=0  MaxVal=1  MeanVal=[0 0 0]'  VarVal="0.01 * (1e-3 * [0.8056    0.5346    0.9000]') .^2"  RepMode=Not repeatable  rawSeed=1  IsInherit=off  SampMode=Discrete  SampTime=1/100  SampFrame=1  DataType=Double  OutComplex=Real  OutputFrames=on
  attitude noise : dspsrcs4/Random Source  SrcType=Gaussian  NormMethod=Ziggurat  CltLength=12  MinVal=0  MaxVal=1  MeanVal=[0 0 0]'  VarVal=[(deg2rad(1))^2 (deg2rad(1))^2 (deg2rad(1))^2]'  RepMode=Not repeatable  rawSeed=1  IsInherit=off  SampMode=Discrete  SampTime=1/100  SampFrame=1  DataType=Double  OutComplex=Real  OutputFrames=on
  output : Outport  OutDataTypeStr=Bus: AHRS
  wires:
  Bus Creator/1 -> output/1
  perfect sensor reading/1 -> Bus Selector/1
  Bus Selector/1 -> Quaternions to Rotation Angles/1  "<quat>"
  Rotation Angles to Quaternions/1 -> Bus Creator/1  "quat"
  Bus Selector/2 -> Add noise1/2  "<gyro_rps>"
  Reshape/1 -> Bus Creator/2  "gyro_rps"
  Quaternions to Rotation Angles/1 -> Add noise2/2
  attitude noise/1 -> Add noise2/1
  Add noise2/1 -> Rotation Angles to Quaternions/1
  angular rate noise/1 -> Add noise1/1
  acceleration noise/1 -> Add noise3/1
  Bus Selector/3 -> Add noise3/2  "<acc_mps2>"
  Reshape1/1 -> Bus Creator/3  "acc_mps2"
  Add noise1/1 -> Reshape/1  "gyro_rps"
  Add noise3/1 -> Reshape1/1  "acc_mps2"

== system formationFlyingBlockset/Add sensor errors/Air Data ==
  perfect sensor reading : Inport  OutDataTypeStr=Bus: SensorBus
  Bus Creator : BusCreator  Inputs=3  OutDataTypeStr=Bus: Airdata
  Bus Selector : BusSelector  OutputSignals=airdata.Tair_K,airdata.pStat_Pa,airdata.qBar_Pa
  Gain : Gain
  Gain1 : Gain
  Gain2 : Gain
  output : Outport  OutDataTypeStr=Bus: Airdata
  wires:
  Gain/1 -> Bus Creator/3  "qBar_Pa"
  Bus Selector/2 -> Gain1/1  "<pStat_Pa>"
  Bus Creator/1 -> output/1
  Gain2/1 -> Bus Creator/1  "Tair_K"
  Gain1/1 -> Bus Creator/2  "pStat_Pa"
  perfect sensor reading/1 -> Bus Selector/1
  Bus Selector/3 -> Gain/1  "<qBar_Pa>"
  Bus Selector/1 -> Gain2/1  "<Tair_K>"

== system formationFlyingBlockset/Add sensor errors/L1 GPS ==
  perfect sensor reading : Inport  OutDataTypeStr=Bus: SensorBus
  Add bias : Sum
  Add noise : Sum
  Add noise1 : Sum
  Bus Creator : BusCreator  Inputs=2  OutDataTypeStr=Bus: GNSSL1
      settings: InheritFromInputs=off
  Bus Selector1 : BusSelector  OutputSignals=gnss_l1.p_ecef_m,gnss_l1.v_ecef_mps
  C\A position noise : dspsrcs4/Random Source  SrcType=Gaussian  NormMethod=Ziggurat  CltLength=12  MinVal=0  MaxVal=1  MeanVal=zeros(3,1)  VarVal=(0.2)^2*ones(3,1)  RepMode=Not repeatable  rawSeed=1  IsInherit=off  SampMode=Discrete  SampTime=1/10  SampFrame=1  DataType=Double  OutComplex=Real  OutputFrames=on
  Doppler velocity noise : dspsrcs4/Random Source  SrcType=Gaussian  NormMethod=Ziggurat  CltLength=12  MinVal=0  MaxVal=1  MeanVal=zeros(3,1)  VarVal=(0.01)^2*ones(3,1)  RepMode=Not repeatable  rawSeed=1  IsInherit=off  SampMode=Discrete  SampTime=1/10  SampFrame=1  DataType=Double  OutComplex=Real  OutputFrames=on
  Integrator : Integrator
  Random walk white noise generator : dspsrcs4/Random Source  SrcType=Uniform  NormMethod=Ziggurat  CltLength=12  MinVal=-1e-6*ones(3,1)  MaxVal=1e-6*ones(3,1)  MeanVal=0  VarVal=1  RepMode=Not repeatable  rawSeed=1  IsInherit=off  SampMode=Discrete  SampTime=1/10  SampFrame=1  DataType=Double  OutComplex=Real  OutputFrames=on
  Reshape : Reshape
  Reshape1 : Reshape
  Scope : Scope
  Scope1 : Scope
  Scope2 : Scope
  output : Outport  OutDataTypeStr=Bus: GNSSL1
  wires:
  Random walk white noise generator/1 -> Integrator/1, Scope2/1
  Add noise/1 -> Add bias/2
  Integrator/1 -> Add bias/1, Scope1/1
  Doppler velocity noise/1 -> Add noise1/2
  C\A position noise/1 -> Add noise/1
  Add noise1/1 -> Reshape1/1  "v_ecef_m"
  Add bias/1 -> Scope/1, Reshape/1  "p_ecef_m"
  Bus Selector1/2 -> Add noise1/1  "<v_ecef_mps>"
  Bus Selector1/1 -> Add noise/2  "<p_ecef_m>"
  Bus Creator/1 -> output/1
  perfect sensor reading/1 -> Bus Selector1/1
  Reshape/1 -> Bus Creator/1  "p_ecef_m"
  Reshape1/1 -> Bus Creator/2  "v_ecef_m"

== system formationFlyingBlockset/Add sensor errors/Optitrack ==
  perfect sensor reading : Inport  OutDataTypeStr=Bus: SensorBus
  Add noise1 : Sum
  Add noise2 : Sum
  Bus Creator : BusCreator  Inputs=2  OutDataTypeStr=Bus: MotionTracker
      settings: InheritFromInputs=off
  Bus Selector : BusSelector  OutputSignals=motiontracker.p_ned_m,motiontracker.v_ned_mps
  Reshape : Reshape
  Reshape1 : Reshape
  position noise : dspsrcs4/Random Source  SrcType=Gaussian  NormMethod=Ziggurat  CltLength=12  MinVal=0  MaxVal=1  MeanVal=zeros(3,1)  VarVal=(0.01)^2*ones(3,1)  RepMode=Not repeatable  rawSeed=1  IsInherit=off  SampMode=Discrete  SampTime=1/10  SampFrame=1  DataType=Double  OutComplex=Real  OutputFrames=on
  velocity noise : dspsrcs4/Random Source  SrcType=Gaussian  NormMethod=Ziggurat  CltLength=12  MinVal=0  MaxVal=1  MeanVal=zeros(3,1)  VarVal=(0.1)^2*ones(3,1)  RepMode=Not repeatable  rawSeed=1  IsInherit=off  SampMode=Discrete  SampTime=1/10  SampFrame=1  DataType=Double  OutComplex=Real  OutputFrames=on
  output : Outport  OutDataTypeStr=Bus: MotionTracker
  wires:
  Add noise1/1 -> Reshape1/1  "delta_v_ecef_mps"
  Add noise2/1 -> Reshape/1  "delta_p_ecef_m"
  perfect sensor reading/1 -> Bus Selector/1
  Bus Creator/1 -> output/1
  Reshape1/1 -> Bus Creator/2  "v_ned_mps"
  Reshape/1 -> Bus Creator/1  "p_ned_m"
  velocity noise/1 -> Add noise1/1
  position noise/1 -> Add noise2/2
  Bus Selector/1 -> Add noise2/1  "<p_ned_m>"
  Bus Selector/2 -> Add noise1/2  "<v_ned_mps>"

== system formationFlyingBlockset/Add sensor errors/Propulsion sensors ==
  perfect sensor reading : Inport  OutDataTypeStr=Bus: SensorBus
  Bus Creator : BusCreator  Inputs=2  OutDataTypeStr=Bus: Enginedata
      settings: InheritFromInputs=off
  I : Constant  Value=0
  U : Constant  Value=0
  output : Outport  OutDataTypeStr=Bus: Enginedata
  wires:
  Bus Creator/1 -> output/1
  I/1 -> Bus Creator/2  "I"
  U/1 -> Bus Creator/1  "U"

== system formationFlyingBlockset/Add sensor errors/RTK DGPS ==
  perfect sensor reading : Inport  OutDataTypeStr=Bus: SensorBus
  Add noise1 : Sum
  Add noise2 : Sum
  Bus Creator : BusCreator  Inputs=2  OutDataTypeStr=Bus: GNSSRTK
      settings: InheritFromInputs=off
  Bus Selector : BusSelector  OutputSignals=gnss_rtk.delta_p_ecef_m,gnss_rtk.delta_v_ecef_mps
  Reshape : Reshape
  Reshape1 : Reshape
  position noise : dspsrcs4/Random Source  SrcType=Gaussian  NormMethod=Ziggurat  CltLength=12  MinVal=0  MaxVal=1  MeanVal=zeros(3,1)  VarVal=(0.01)^2*ones(3,1)  RepMode=Not repeatable  rawSeed=1  IsInherit=off  SampMode=Discrete  SampTime=1/10  SampFrame=1  DataType=Double  OutComplex=Real  OutputFrames=on
  velocity noise : dspsrcs4/Random Source  SrcType=Gaussian  NormMethod=Ziggurat  CltLength=12  MinVal=0  MaxVal=1  MeanVal=zeros(3,1)  VarVal=(0.1)^2*ones(3,1)  RepMode=Not repeatable  rawSeed=1  IsInherit=off  SampMode=Discrete  SampTime=1/10  SampFrame=1  DataType=Double  OutComplex=Real  OutputFrames=on
  output : Outport  OutDataTypeStr=Bus: GNSSRTK
  wires:
  Bus Selector/2 -> Add noise1/2  "<delta_v_ecef_mps>"
  Bus Selector/1 -> Add noise2/1  "<delta_p_ecef_m>"
  position noise/1 -> Add noise2/2
  velocity noise/1 -> Add noise1/1
  Reshape/1 -> Bus Creator/1  "delta_p_ecef_m"
  Reshape1/1 -> Bus Creator/2  "delta_v_ecef_mps"
  Bus Creator/1 -> output/1
  perfect sensor reading/1 -> Bus Selector/1
  Add noise2/1 -> Reshape/1  "delta_p_ecef_m"
  Add noise1/1 -> Reshape1/1  "delta_v_ecef_mps"

== system formationFlyingBlockset/Add sensor errors/Radio distance sensor ==
  perfect sensor reading : Inport  OutDataTypeStr=Bus: SensorBus
  Add noise : Sum
  Bus Creator : BusCreator  Inputs=1  OutDataTypeStr=Bus: Radiodistance
      settings: InheritFromInputs=off
  Bus Selector1 : BusSelector  OutputSignals=radiodistance.r
  Random Source : dspsrcs4/Random Source  SrcType=Gaussian  NormMethod=Ziggurat  CltLength=12  MinVal=-0.3  MaxVal=0.3  MeanVal=0  VarVal=3e-4  RepMode=Not repeatable  rawSeed=1  IsInherit=off  SampMode=Discrete  SampTime=0.01  SampFrame=1  DataType=Double  OutComplex=Real  OutputFrames=on
  vector norm : uavsimBlockset_VectorNorm/vector norm
  output : Outport  OutDataTypeStr=Bus: Radiodistance
  wires:
  Random Source/1 -> Add noise/1
  Add noise/1 -> Bus Creator/1  "r"
  vector norm/1 -> Add noise/2
  Bus Creator/1 -> output/1
  Bus Selector1/1 -> vector norm/1  "<r>"
  perfect sensor reading/1 -> Bus Selector1/1

== system formationFlyingBlockset/Add sensor errors/Wind angle sensors ==
  perfect sensor reading : Inport  OutDataTypeStr=Bus: SensorBus
  Bus Creator : BusCreator  Inputs=2  OutDataTypeStr=Bus: WindAngles
  Bus Selector : BusSelector  OutputSignals=windangles.alpha_rad,windangles.beta_rad
  Gain : Gain
  Gain1 : Gain
  output : Outport  OutDataTypeStr=Bus: WindAngles
  wires:
  Gain1/1 -> Bus Creator/2  "beta_rad"
  Gain/1 -> Bus Creator/1  "alpha_rad"
  Bus Selector/2 -> Gain1/1  "<beta_rad>"
  Bus Selector/1 -> Gain/1  "<alpha_rad>"
  Bus Creator/1 -> output/1
  perfect sensor reading/1 -> Bus Selector/1
